simulink library "CRYP_TM_MASTER"  (Simulink 8.6)
settings: Solver=ode45  StartTime=0.0  StopTime=10.0  RelTol=1e-3
libraries: cdsEpicsOut x44, cdsTP x11, cdsFilt x5, cdsFiltCtrl x4, cdsFunctionCall x4, CRYP_TM_MASTER x3, QPD x2, VIS_LIB x1, cdsMuxMatrix x1
(part 2 of 2)

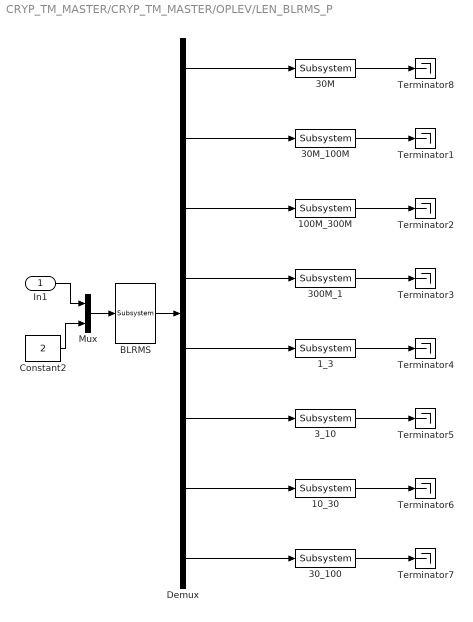
== system CRYP_TM_MASTER/CRYP_TM_MASTER/OPLEV/LEN_BLRMS_P ==
  In1 : Inport
  100M_300M : cdsEpicsOut/Subsystem  Tag=cdsEpicsOutput  Description=|
      | Purpose:                                          
      | Output a FE signal to an EPICS channel.           
      |                                                   
      | Operation:                                        
      | Takes input value and passes it to EPICS record.  
      |                                                   
      | Usage:                                            
      | Name the part with the desired EPICS rrecord name.
      settings: AttributesFormatString=%<Tag>
  10_30 : cdsEpicsOut/Subsystem  Tag=cdsEpicsOutput  Description=|
      | Purpose:                                          
      | Output a FE signal to an EPICS channel.           
      |                                                   
      | Operation:                                        
      | Takes input value and passes it to EPICS record.  
      |                                                   
      | Usage:                                            
      | Name the part with the desired EPICS rrecord name.
      settings: AttributesFormatString=%<Tag>
  1_3 : cdsEpicsOut/Subsystem  Tag=cdsEpicsOutput  Description=|
      | Purpose:                                          
      | Output a FE signal to an EPICS channel.           
      |                                                   
      | Operation:                                        
      | Takes input value and passes it to EPICS record.  
      |                                                   
      | Usage:                                            
      | Name the part with the desired EPICS rrecord name.
      settings: AttributesFormatString=%<Tag>
  300M_1 : cdsEpicsOut/Subsystem  Tag=cdsEpicsOutput  Description=|
      | Purpose:                                          
      | Output a FE signal to an EPICS channel.           
      |                                                   
      | Operation:                                        
      | Takes input value and passes it to EPICS record.  
      |                                                   
      | Usage:                                            
      | Name the part with the desired EPICS rrecord name.
      settings: AttributesFormatString=%<Tag>
  30M : cdsEpicsOut/Subsystem  Tag=cdsEpicsOutput  Description=|
      | Purpose:                                          
      | Output a FE signal to an EPICS channel.           
      |                                                   
      | Operation:                                        
      | Takes input value and passes it to EPICS record.  
      |                                                   
      | Usage:                                            
      | Name the part with the desired EPICS rrecord name.
      settings: AttributesFormatString=%<Tag>
  30M_100M : cdsEpicsOut/Subsystem  Tag=cdsEpicsOutput  Description=|
      | Purpose:                                          
      | Output a FE signal to an EPICS channel.           
      |                                                   
      | Operation:                                        
      | Takes input value and passes it to EPICS record.  
      |                                                   
      | Usage:                                            
      | Name the part with the desired EPICS rrecord name.
      settings: AttributesFormatString=%<Tag>
  30_100 : cdsEpicsOut/Subsystem  Tag=cdsEpicsOutput  Description=|
      | Purpose:                                          
      | Output a FE signal to an EPICS channel.           
      |                                                   
      | Operation:                                        
      | Takes input value and passes it to EPICS record.  
      |                                                   
      | Usage:                                            
      | Name the part with the desired EPICS rrecord name.
      settings: AttributesFormatString=%<Tag>
  3_10 : cdsEpicsOut/Subsystem  Tag=cdsEpicsOutput  Description=|
      | Purpose:                                          
      | Output a FE signal to an EPICS channel.           
      |                                                   
      | Operation:                                        
      | Takes input value and passes it to EPICS record.  
      |                                                   
      | Usage:                                            
      | Name the part with the desired EPICS rrecord name.
      settings: AttributesFormatString=%<Tag>
  BLRMS : cdsFunctionCall/Subsystem  Tag=cdsFunctionCall  Description=inline BLRMS /opt/rtcds/userapps/release/cds/common/src/BLRMSFILTER.c
      settings: AttributesFormatString=%<Tag>\n%<Description>
  Constant2 : Constant  Value=2
  Demux : Demux  Outputs=8
  Mux : Mux  Inputs=2
  Terminator{1..8} (8 alike) : Terminator
  wires:
  BLRMS/1 -> Demux/1
  Mux/1 -> BLRMS/1
  In1/1 -> Mux/1
  Demux/1 -> 30M/1
  Demux/2 -> 30M_100M/1
  Demux/3 -> 100M_300M/1
  Demux/4 -> 300M_1/1
  Demux/5 -> 1_3/1
  Demux/6 -> 3_10/1
  Demux/7 -> 10_30/1
  Demux/8 -> 30_100/1
  30M/1 -> Terminator8/1
  30M_100M/1 -> Terminator1/1
  100M_300M/1 -> Terminator2/1
  300M_1/1 -> Terminator3/1
  1_3/1 -> Terminator4/1
  3_10/1 -> Terminator5/1
  10_30/1 -> Terminator6/1
  30_100/1 -> Terminator7/1
  Constant2/1 -> Mux/2

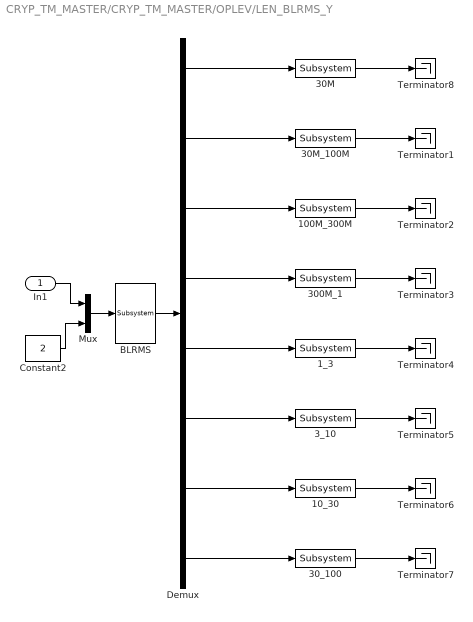
== system CRYP_TM_MASTER/CRYP_TM_MASTER/OPLEV/LEN_BLRMS_Y ==
  In1 : Inport
  100M_300M : cdsEpicsOut/Subsystem  Tag=cdsEpicsOutput  Description=|
      | Purpose:                                          
      | Output a FE signal to an EPICS channel.           
      |                                                   
      | Operation:                                        
      | Takes input value and passes it to EPICS record.  
      |                                                   
      | Usage:                                            
      | Name the part with the desired EPICS rrecord name.
      settings: AttributesFormatString=%<Tag>
  10_30 : cdsEpicsOut/Subsystem  Tag=cdsEpicsOutput  Description=|
      | Purpose:                                          
      | Output a FE signal to an EPICS channel.           
      |                                                   
      | Operation:                                        
      | Takes input value and passes it to EPICS record.  
      |                                                   
      | Usage:                                            
      | Name the part with the desired EPICS rrecord name.
      settings: AttributesFormatString=%<Tag>
  1_3 : cdsEpicsOut/Subsystem  Tag=cdsEpicsOutput  Description=|
      | Purpose:                                          
      | Output a FE signal to an EPICS channel.           
      |                                                   
      | Operation:                                        
      | Takes input value and passes it to EPICS record.  
      |                                                   
      | Usage:                                            
      | Name the part with the desired EPICS rrecord name.
      settings: AttributesFormatString=%<Tag>
  300M_1 : cdsEpicsOut/Subsystem  Tag=cdsEpicsOutput  Description=|
      | Purpose:                                          
      | Output a FE signal to an EPICS channel.           
      |                                                   
      | Operation:                                        
      | Takes input value and passes it to EPICS record.  
      |                                                   
      | Usage:                                            
      | Name the part with the desired EPICS rrecord name.
      settings: AttributesFormatString=%<Tag>
  30M : cdsEpicsOut/Subsystem  Tag=cdsEpicsOutput  Description=|
      | Purpose:                                          
      | Output a FE signal to an EPICS channel.           
      |                                                   
      | Operation:                                        
      | Takes input value and passes it to EPICS record.  
      |                                                   
      | Usage:                                            
      | Name the part with the desired EPICS rrecord name.
      settings: AttributesFormatString=%<Tag>
  30M_100M : cdsEpicsOut/Subsystem  Tag=cdsEpicsOutput  Description=|
      | Purpose:                                          
      | Output a FE signal to an EPICS channel.           
      |                                                   
      | Operation:                                        
      | Takes input value and passes it to EPICS record.  
      |                                                   
      | Usage:                                            
      | Name the part with the desired EPICS rrecord name.
      settings: AttributesFormatString=%<Tag>
  30_100 : cdsEpicsOut/Subsystem  Tag=cdsEpicsOutput  Description=|
      | Purpose:                                          
      | Output a FE signal to an EPICS channel.           
      |                                                   
      | Operation:                                        
      | Takes input value and passes it to EPICS record.  
      |                                                   
      | Usage:                                            
      | Name the part with the desired EPICS rrecord name.
      settings: AttributesFormatString=%<Tag>
  3_10 : cdsEpicsOut/Subsystem  Tag=cdsEpicsOutput  Description=|
      | Purpose:                                          
      | Output a FE signal to an EPICS channel.           
      |                                                   
      | Operation:                                        
      | Takes input value and passes it to EPICS record.  
      |                                                   
      | Usage:                                            
      | Name the part with the desired EPICS rrecord name.
      settings: AttributesFormatString=%<Tag>
  BLRMS : cdsFunctionCall/Subsystem  Tag=cdsFunctionCall  Description=inline BLRMS /opt/rtcds/userapps/release/cds/common/src/BLRMSFILTER.c
      settings: AttributesFormatString=%<Tag>\n%<Description>
  Constant2 : Constant  Value=2
  Demux : Demux  Outputs=8
  Mux : Mux  Inputs=2
  Terminator{1..8} (8 alike) : Terminator
  wires:
  BLRMS/1 -> Demux/1
  Mux/1 -> BLRMS/1
  In1/1 -> Mux/1
  Demux/1 -> 30M/1
  Demux/2 -> 30M_100M/1
  Demux/3 -> 100M_300M/1
  Demux/4 -> 300M_1/1
  Demux/5 -> 1_3/1
  Demux/6 -> 3_10/1
  Demux/7 -> 10_30/1
  Demux/8 -> 30_100/1
  30M/1 -> Terminator8/1
  30M_100M/1 -> Terminator1/1
  100M_300M/1 -> Terminator2/1
  300M_1/1 -> Terminator3/1
  1_3/1 -> Terminator4/1
  3_10/1 -> Terminator5/1
  10_30/1 -> Terminator6/1
  30_100/1 -> Terminator7/1
  Constant2/1 -> Mux/2

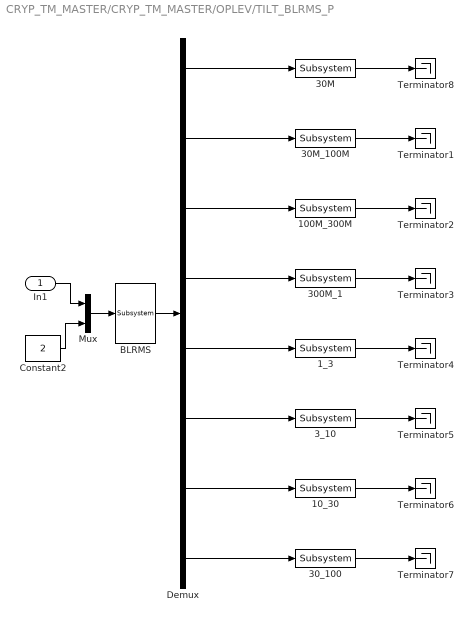
== system CRYP_TM_MASTER/CRYP_TM_MASTER/OPLEV/TILT_BLRMS_P ==
  In1 : Inport
  100M_300M : cdsEpicsOut/Subsystem  Tag=cdsEpicsOutput  Description=|
      | Purpose:                                          
      | Output a FE signal to an EPICS channel.           
      |                                                   
      | Operation:                                        
      | Takes input value and passes it to EPICS record.  
      |                                                   
      | Usage:                                            
      | Name the part with the desired EPICS rrecord name.
      settings: AttributesFormatString=%<Tag>
  10_30 : cdsEpicsOut/Subsystem  Tag=cdsEpicsOutput  Description=|
      | Purpose:                                          
      | Output a FE signal to an EPICS channel.           
      |                                                   
      | Operation:                                        
      | Takes input value and passes it to EPICS record.  
      |                                                   
      | Usage:                                            
      | Name the part with the desired EPICS rrecord name.
      settings: AttributesFormatString=%<Tag>
  1_3 : cdsEpicsOut/Subsystem  Tag=cdsEpicsOutput  Description=|
      | Purpose:                                          
      | Output a FE signal to an EPICS channel.           
      |                                                   
      | Operation:                                        
      | Takes input value and passes it to EPICS record.  
      |                                                   
      | Usage:                                            
      | Name the part with the desired EPICS rrecord name.
      settings: AttributesFormatString=%<Tag>
  300M_1 : cdsEpicsOut/Subsystem  Tag=cdsEpicsOutput  Description=|
      | Purpose:                                          
      | Output a FE signal to an EPICS channel.           
      |                                                   
      | Operation:                                        
      | Takes input value and passes it to EPICS record.  
      |                                                   
      | Usage:                                            
      | Name the part with the desired EPICS rrecord name.
      settings: AttributesFormatString=%<Tag>
  30M : cdsEpicsOut/Subsystem  Tag=cdsEpicsOutput  Description=|
      | Purpose:                                          
      | Output a FE signal to an EPICS channel.           
      |                                                   
      | Operation:                                        
      | Takes input value and passes it to EPICS record.  
      |                                                   
      | Usage:                                            
      | Name the part with the desired EPICS rrecord name.
      settings: AttributesFormatString=%<Tag>
  30M_100M : cdsEpicsOut/Subsystem  Tag=cdsEpicsOutput  Description=|
      | Purpose:                                          
      | Output a FE signal to an EPICS channel.           
      |                                                   
      | Operation:                                        
      | Takes input value and passes it to EPICS record.  
      |                                                   
      | Usage:                                            
      | Name the part with the desired EPICS rrecord name.
      settings: AttributesFormatString=%<Tag>
  30_100 : cdsEpicsOut/Subsystem  Tag=cdsEpicsOutput  Description=|
      | Purpose:                                          
      | Output a FE signal to an EPICS channel.           
      |                                                   
      | Operation:                                        
      | Takes input value and passes it to EPICS record.  
      |                                                   
      | Usage:                                            
      | Name the part with the desired EPICS rrecord name.
      settings: AttributesFormatString=%<Tag>
  3_10 : cdsEpicsOut/Subsystem  Tag=cdsEpicsOutput  Description=|
      | Purpose:                                          
      | Output a FE signal to an EPICS channel.           
      |                                                   
      | Operation:                                        
      | Takes input value and passes it to EPICS record.  
      |                                                   
      | Usage:                                            
      | Name the part with the desired EPICS rrecord name.
      settings: AttributesFormatString=%<Tag>
  BLRMS : cdsFunctionCall/Subsystem  Tag=cdsFunctionCall  Description=inline BLRMS /opt/rtcds/userapps/release/cds/common/src/BLRMSFILTER.c
      settings: AttributesFormatString=%<Tag>\n%<Description>
  Constant2 : Constant  Value=2
  Demux : Demux  Outputs=8
  Mux : Mux  Inputs=2
  Terminator{1..8} (8 alike) : Terminator
  wires:
  BLRMS/1 -> Demux/1
  Mux/1 -> BLRMS/1
  In1/1 -> Mux/1
  Demux/1 -> 30M/1
  Demux/2 -> 30M_100M/1
  Demux/3 -> 100M_300M/1
  Demux/4 -> 300M_1/1
  Demux/5 -> 1_3/1
  Demux/6 -> 3_10/1
  Demux/7 -> 10_30/1
  Demux/8 -> 30_100/1
  30M/1 -> Terminator8/1
  30M_100M/1 -> Terminator1/1
  100M_300M/1 -> Terminator2/1
  300M_1/1 -> Terminator3/1
  1_3/1 -> Terminator4/1
  3_10/1 -> Terminator5/1
  10_30/1 -> Terminator6/1
  30_100/1 -> Terminator7/1
  Constant2/1 -> Mux/2

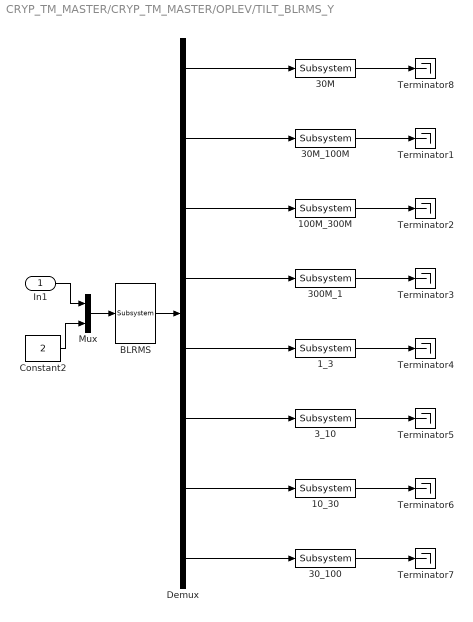
== system CRYP_TM_MASTER/CRYP_TM_MASTER/OPLEV/TILT_BLRMS_Y ==
  In1 : Inport
  100M_300M : cdsEpicsOut/Subsystem  Tag=cdsEpicsOutput  Description=|
      | Purpose:                                          
      | Output a FE signal to an EPICS channel.           
      |                                                   
      | Operation:                                        
      | Takes input value and passes it to EPICS record.  
      |                                                   
      | Usage:                                            
      | Name the part with the desired EPICS rrecord name.
      settings: AttributesFormatString=%<Tag>
  10_30 : cdsEpicsOut/Subsystem  Tag=cdsEpicsOutput  Description=|
      | Purpose:                                          
      | Output a FE signal to an EPICS channel.           
      |                                                   
      | Operation:                                        
      | Takes input value and passes it to EPICS record.  
      |                                                   
      | Usage:                                            
      | Name the part with the desired EPICS rrecord name.
      settings: AttributesFormatString=%<Tag>
  1_3 : cdsEpicsOut/Subsystem  Tag=cdsEpicsOutput  Description=|
      | Purpose:                                          
      | Output a FE signal to an EPICS channel.           
      |                                                   
      | Operation:                                        
      | Takes input value and passes it to EPICS record.  
      |                                                   
      | Usage:                                            
      | Name the part with the desired EPICS rrecord name.
      settings: AttributesFormatString=%<Tag>
  300M_1 : cdsEpicsOut/Subsystem  Tag=cdsEpicsOutput  Description=|
      | Purpose:                                          
      | Output a FE signal to an EPICS channel.           
      |                                                   
      | Operation:                                        
      | Takes input value and passes it to EPICS record.  
      |                                                   
      | Usage:                                            
      | Name the part with the desired EPICS rrecord name.
      settings: AttributesFormatString=%<Tag>
  30M : cdsEpicsOut/Subsystem  Tag=cdsEpicsOutput  Description=|
      | Purpose:                                          
      | Output a FE signal to an EPICS channel.           
      |                                                   
      | Operation:                                        
      | Takes input value and passes it to EPICS record.  
      |                                                   
      | Usage:                                            
      | Name the part with the desired EPICS rrecord name.
      settings: AttributesFormatString=%<Tag>
  30M_100M : cdsEpicsOut/Subsystem  Tag=cdsEpicsOutput  Description=|
      | Purpose:                                          
      | Output a FE signal to an EPICS channel.           
      |                                                   
      | Operation:                                        
      | Takes input value and passes it to EPICS record.  
      |                                                   
      | Usage:                                            
      | Name the part with the desired EPICS rrecord name.
      settings: AttributesFormatString=%<Tag>
  30_100 : cdsEpicsOut/Subsystem  Tag=cdsEpicsOutput  Description=|
      | Purpose:                                          
      | Output a FE signal to an EPICS channel.           
      |                                                   
      | Operation:                                        
      | Takes input value and passes it to EPICS record.  
      |                                                   
      | Usage:                                            
      | Name the part with the desired EPICS rrecord name.
      settings: AttributesFormatString=%<Tag>
  3_10 : cdsEpicsOut/Subsystem  Tag=cdsEpicsOutput  Description=|
      | Purpose:                                          
      | Output a FE signal to an EPICS channel.           
      |                                                   
      | Operation:                                        
      | Takes input value and passes it to EPICS record.  
      |                                                   
      | Usage:                                            
      | Name the part with the desired EPICS rrecord name.
      settings: AttributesFormatString=%<Tag>
  BLRMS : cdsFunctionCall/Subsystem  Tag=cdsFunctionCall  Description=inline BLRMS /opt/rtcds/userapps/release/cds/common/src/BLRMSFILTER.c
      settings: AttributesFormatString=%<Tag>\n%<Description>
  Constant2 : Constant  Value=2
  Demux : Demux  Outputs=8
  Mux : Mux  Inputs=2
  Terminator{1..8} (8 alike) : Terminator
  wires:
  BLRMS/1 -> Demux/1
  Mux/1 -> BLRMS/1
  In1/1 -> Mux/1
  Demux/1 -> 30M/1
  Demux/2 -> 30M_100M/1
  Demux/3 -> 100M_300M/1
  Demux/4 -> 300M_1/1
  Demux/5 -> 1_3/1
  Demux/6 -> 3_10/1
  Demux/7 -> 10_30/1
  Demux/8 -> 30_100/1
  30M/1 -> Terminator8/1
  30M_100M/1 -> Terminator1/1
  100M_300M/1 -> Terminator2/1
  300M_1/1 -> Terminator3/1
  1_3/1 -> Terminator4/1
  3_10/1 -> Terminator5/1
  10_30/1 -> Terminator6/1
  30_100/1 -> Terminator7/1
  Constant2/1 -> Mux/2
